simulink model "Simulink_AcraV3"  (R2018a)
settings: Solver=VariableStepAuto  StartTime=0.0  StopTime=total_time  FixedStep=step  RelTol=1e-3  AbsTol=1e-3  EnableMultiTasking=on
values from neighbouring files (symbols this model uses):
  C1 = 35/1000    (= 0.035)    [ACRA_simulink.m]
  C2 = 32/1000    (= 0.032)    [ACRA_simulink.m]
  K_ow = 20    [ACRA_simulink.m]
  K_peep = 25    [ACRA_simulink.m]
  Kv1 = 30    [ACRA_simulink.m]
  Kv2 = 40    [ACRA_simulink.m]
  PEEP_v1 = 5    [ACRA_simulink.m]
  PEEP_v2 = 7    [ACRA_simulink.m]
  R1 = 5    [ACRA_simulink.m]
  R2 = 7    [ACRA_simulink.m]
  R_vent = 1.5    [ACRA_simulink.m]
libraries: sh_lib x23, fl_lib x16, nesl_utility x9, sdl_lib x4
settings Model: Creator=Pedro  LastModifiedBy=Pedro
settings SolverCC: AutoScaleAbsTol=off  ZeroCrossAlgorithm=Adaptive
settings DataIOCC: LimitDataPoints=on  MaxDataPoints=10000
settings OptimizationCC: LifeSpan=inf
settings DebuggingCC: IgnoredZcDiagnostic=none  AllowSymbolicDim=off  SFUnexpectedBacktrackingDiag=warning  SFNoUnconditionalDefaultTransitionDiag=warning  SFExecutionAtInitializationDiag=none
settings CodeAppCC: StateflowObjectComments=on
settings GRTTargetCC: TargetLangStandard=C89/C90 (ANSI)  GeneratePreprocessorConditionals=Disable all
settings ConfigComp: CovMetricSettings=dw  CovHtmlReporting=on  CovSaveCumulativeToWorkspaceVar=on  CovSaveSingleToWorkspaceVar=on  CovExternalEMLEnable=off  CovSFcnEnable=off
settings SimscapeCC: SimscapeLogType=all  SimscapeLogDataHistory=10000

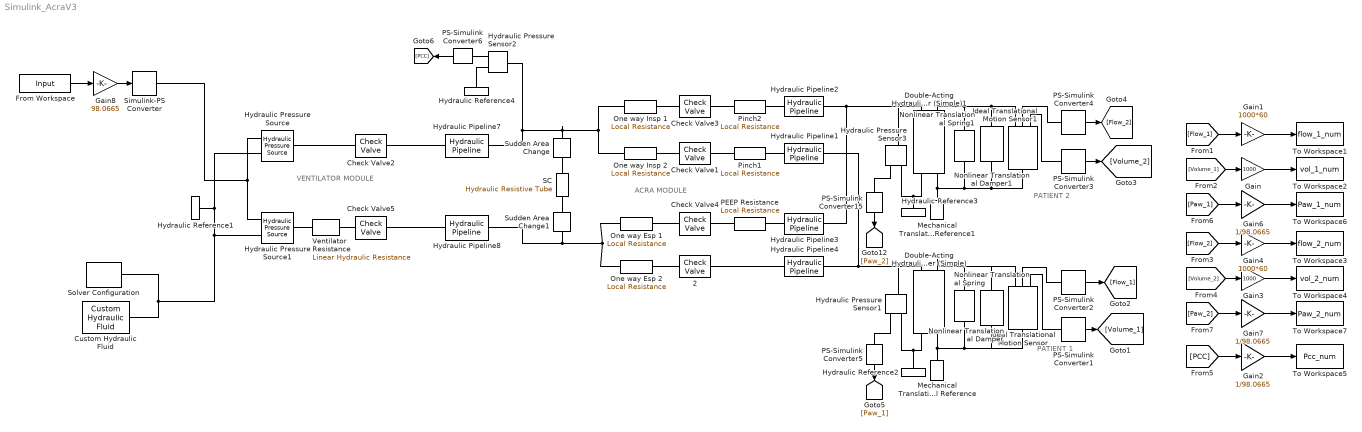
== system Simulink_AcraV3 ==
  note: PATIENT 2
  note: PATIENT 1
  note: VENTILATOR
      | MODULE
  note: ACRA MODULE
  " 2" : sh_lib/Valves/Directional Valves/Check Valve  area_max=5 cm^2  pres_crack=1 Pa  pres_max=10 Pa  C_d=1  A_leak=1e-12 cm^2  lam_spec=1  B_lam=0.999  Re_cr=12  dynamic=1  tau=0.05 s  area_init=1e-12 m^2
      settings: SourceProductName=Simscape Fluids  SourceProductBaseCode=SH
  Check Valve1 : sh_lib/Valves/Directional Valves/Check Valve  area_max=5 cm^2  pres_crack=1 Pa  pres_max=10 Pa  C_d=1  A_leak=1e-12 mm^2  lam_spec=2  B_lam=0.999  Re_cr=1000  dynamic=1  tau=0.05 s  area_init=1e-12 m^2
      settings: SourceProductName=Simscape Fluids  SourceProductBaseCode=SH
  Check Valve2 : sh_lib/Valves/Directional Valves/Check Valve  area_max=5 cm^2  pres_crack=1 Pa  pres_max=10 Pa  C_d=1  A_leak=1e-12 mm^2  lam_spec=2  B_lam=0.999  Re_cr=1000  dynamic=1  tau=0.05 s  area_init=1e-12 m^2
      settings: SourceProductName=Simscape Fluids  SourceProductBaseCode=SH
  Check Valve3 : sh_lib/Valves/Directional Valves/Check Valve  area_max=5 cm^2  pres_crack=1 Pa  pres_max=10 Pa  C_d=1  A_leak=1e-12 mm^2  lam_spec=2  B_lam=0.999  Re_cr=1000  dynamic=1  tau=0.05 s  area_init=1e-12 m^2
      settings: SourceProductName=Simscape Fluids  SourceProductBaseCode=SH
  Check Valve4 : sh_lib/Valves/Directional Valves/Check Valve  area_max=1 cm^2  pres_crack=(PEEP_v2-PEEP_v1+0.01)*98 Pa  pres_max=(PEEP_v2-PEEP_v1+0.01)*98.1 Pa  C_d=1  A_leak=1e-12 mm^2  lam_spec=2  B_lam=0.999  Re_cr=4000  dynamic=1  tau=0.05 s  area_init=1e-12 m^2
      settings: SourceProductName=Simscape Fluids  SourceProductBaseCode=SH
  Check Valve5 : sh_lib/Valves/Directional Valves/Check Valve  area_max=0.8 cm^2  pres_crack=0.01*98 Pa  pres_max=0.2*98 Pa  C_d=1  A_leak=1e-12 mm^2  lam_spec=2  B_lam=0.999  Re_cr=4000  dynamic=1  tau=0.1 s  area_init=1e-12 m^2
      settings: SourceProductName=Simscape Fluids  SourceProductBaseCode=SH
  Custom Hydraulic Fluid : fl_lib/Hydraulic/Hydraulic Utilities/Custom Hydraulic Fluid  density=1.225 kg/m^3  viscosity_kin=1.5e-5 m^2/s  bulk=142 kPa  alpha=0.005  range_error=2
      settings: SourceProductName=Foundation Library
  Double-Acting Hydraulic Cylinder (Simple) : sh_lib/Hydraulic Cylinders/Double-Acting Hydraulic Cylinder (Simple)  area_A=1 m^2  area_B=1 m^2  stroke=1 m  init_pos=0 m  penetr_coeff=1e12 s*N/m^2  or=1
      settings: SourceProductName=Simscape Fluids  SourceProductBaseCode=SH
  Double-Acting Hydraulic Cylinder (Simple)1 : sh_lib/Hydraulic Cylinders/Double-Acting Hydraulic Cylinder (Simple)  area_A=1 m^2  area_B=1 m^2  stroke=1 m  init_pos=0 m  penetr_coeff=1e12 s*N/m^2  or=1
      settings: SourceProductName=Simscape Fluids  SourceProductBaseCode=SH
  From Workspace : FromWorkspace  VariableName=Input  OutDataTypeStr=double  SampleTime=0
  Gain : Gain  Gain=1000
  Gain1 : Gain  Gain=1000*60
  Gain2 : Gain  Gain=1/98.0665
  Gain3 : Gain  Gain=1000
  Gain4 : Gain  Gain=1000*60
  Gain6 : Gain  Gain=1/98.0665
  Gain7 : Gain  Gain=1/98.0665
  Gain8 : Gain  Gain=98.0665
  Hydraulic Pipeline{1..4,7..8} (6 alike) : sh_lib/Pipelines/Hydraulic Pipeline  cs_type=1  d_in=20 mm  area=1e-4 m^2  D_h=1.12e-2 m  s_factor=64  length=1 m  length_ad=0.1 m  roughness=0.2 mm  Re_lam=2000  Re_turb=4000  wall_type=2  pr_r_coef=4e-8 m/Pa  time_const=0.01 s  k_sh=1.4  initial_pressure=0 Pa
      settings: SourceProductName=Simscape Fluids  SourceProductBaseCode=SH
  Hydraulic Pressure Sensor1 : fl_lib/Hydraulic/Hydraulic Sensors/Hydraulic Pressure Sensor
      settings: SourceProductName=Simscape
  Hydraulic Pressure Sensor2 : fl_lib/Hydraulic/Hydraulic Sensors/Hydraulic Pressure Sensor
      settings: SourceProductName=Simscape
  Hydraulic Pressure Sensor3 : fl_lib/Hydraulic/Hydraulic Sensors/Hydraulic Pressure Sensor
      settings: SourceProductName=Simscape
  Hydraulic Pressure Source : fl_lib/Hydraulic/Hydraulic Sources/Hydraulic Pressure Source
      settings: SourceProductName=Simscape  SourceProductBaseCode=SS
  Hydraulic Pressure Source1 : fl_lib/Hydraulic/Hydraulic Sources/Hydraulic Pressure Source
      settings: SourceProductName=Simscape  SourceProductBaseCode=SS
  Hydraulic Reference{1..4} (4 alike) : fl_lib/Hydraulic/Hydraulic Elements/Hydraulic Reference
      settings: SourceProductName=Foundation Library
  Ideal Translational Motion Sensor : fl_lib/Mechanical/Mechanical Sensors/Ideal Translational Motion Sensor  offset=0 m
  Ideal Translational Motion Sensor1 : fl_lib/Mechanical/Mechanical Sensors/Ideal Translational Motion Sensor  offset=0 m
  Mechanical Translational Reference : fl_lib/Mechanical/Translational Elements/Mechanical Translational Reference
  Mechanical Translational Reference1 : fl_lib/Mechanical/Translational Elements/Mechanical Translational Reference
  Nonlinear Translational Damper : sdl_lib/Couplings & Drives/Springs & Dampers/Nonlinear Translational Damper  parameterization=1  symmetry=1  coefficient_vector=[R1*98*1000, 0, 0, 0, 0] N/(m/s)  extension_coefficient_vector=[10, 0, 1, 0, .1] N/(m/s)  contraction_coefficient_vector=[100, -1, 10, 0, 0] N/(m/s)  velocity_vector=[-1, -.5, -.3, -.1, .1, .3, .5, 1] m/s  force_vector=[-100, -40, -20, -5, 5, 20, 40, 100] N  interp_method=simscape.enum.interpolation.linear  extrap_method=simscape.enum.extrapolation.linear
      settings: SourceProductName=Simscape Driveline  SourceProductBaseCode=LD
  Nonlinear Translational Damper1 : sdl_lib/Couplings & Drives/Springs & Dampers/Nonlinear Translational Damper  parameterization=1  symmetry=1  coefficient_vector=[R2*98*1000, 0, 0, 0, 0] N/(m/s)  extension_coefficient_vector=[10, 0, 1, 0, .1] N/(m/s)  contraction_coefficient_vector=[100, -1, 10, 0, 0] N/(m/s)  velocity_vector=[-1, -.5, -.3, -.1, .1, .3, .5, 1] m/s  force_vector=[-100, -40, -20, -5, 5, 20, 40, 100] N  interp_method=simscape.enum.interpolation.linear  extrap_method=simscape.enum.extrapolation.linear
      settings: SourceProductName=Simscape Driveline  SourceProductBaseCode=LD
  Nonlinear Translational Spring : sdl_lib/Couplings & Drives/Springs & Dampers/Nonlinear Translational Spring  parameterization=1  symmetry=1  coefficient_vector=[1000*98.0665/C1, 0, 0, 0, 0] N/m  tension_coefficient_vector=[100, 0, 10, 0, 1] N/m  compression_coefficient_vector=[1000, -10, 100, 0, 0] N/m  deformation_vector=[0,100,200,400,600,800,1000,1200]*1/1000 mm  force_vector=[0,345,780,1340,1530,1600,1710,2900]*1.1 N  interp_method=simscape.enum.interpolation.linear  extrap_method=simscape.enum.extrapolation.linear  x_specify=off  x_priority=High  x=0 m  x_nominal_specify=off  x_nominal_unit=m  x_nominal_value=1
      settings: SourceProductName=Simscape Driveline  SourceProductBaseCode=LD
  Nonlinear Translational Spring1 : sdl_lib/Couplings & Drives/Springs & Dampers/Nonlinear Translational Spring  parameterization=1  symmetry=1  coefficient_vector=[1000*98.0665/C2, 0, 0, 0, 0] N/m  tension_coefficient_vector=[100, 0, 10, 0, 1] N/m  compression_coefficient_vector=[1000, -10, 100, 0, 0] N/m  deformation_vector=[0,100,200,400,600,800,1000,1200]*1/1000 mm  force_vector=[0,345,780,1340,1530,1600,1710,2900]*1.1 N  interp_method=simscape.enum.interpolation.linear  extrap_method=simscape.enum.extrapolation.linear  x_specify=off  x_priority=High  x=0 m  x_nominal_specify=off  x_nominal_unit=m  x_nominal_value=1
      settings: SourceProductName=Simscape Driveline  SourceProductBaseCode=LD
  One way Esp 1 : sh_lib/Local Hydraulic Resistances/Local Resistance  area=0.000198456 m^2  mdl_type=2  kp_d=40  kp_r=40  lam_spec=2  B_lam=0.999  Re_cr=1000  Re_vec=[-10000 , 0, 10000]  loss_coeff_vec=[1,1,1]*(K_ow)  interp_method=1  extrap_method=2  flow_rate_threshold=1e-6 m^3/s  flow_rate_specify=off  flow_rate_priority=None  flow_rate=0 m^3/s  flow_rate_nominal_specify=off  flow_rate_nominal_unit=m^3/s  flow_rate_nominal_value=1  pressure_drop_specify=off  pressure_drop_priority=None  pressure_drop=0 Pa  pressure_drop_nominal_specify=off  pressure_drop_nominal_unit=Pa  pressure_drop_nominal_value=1
      settings: SourceProductName=Simscape Fluids  SourceProductBaseCode=SH
  One way Esp 2 : sh_lib/Local Hydraulic Resistances/Local Resistance  area=0.000198456 m^2  mdl_type=2  kp_d=40  kp_r=40  lam_spec=2  B_lam=0.999  Re_cr=1000  Re_vec=[-10000 , 0, 10000]  loss_coeff_vec=[1,1,1]*K_ow  interp_method=1  extrap_method=2  flow_rate_threshold=1e-6 m^3/s  flow_rate_specify=off  flow_rate_priority=None  flow_rate=0 m^3/s  flow_rate_nominal_specify=off  flow_rate_nominal_unit=m^3/s  flow_rate_nominal_value=1  pressure_drop_specify=off  pressure_drop_priority=None  pressure_drop=0 Pa  pressure_drop_nominal_specify=off  pressure_drop_nominal_unit=Pa  pressure_drop_nominal_value=1
      settings: SourceProductName=Simscape Fluids  SourceProductBaseCode=SH
  One way Insp 1 : sh_lib/Local Hydraulic Resistances/Local Resistance  area=0.000198456 m^2  mdl_type=2  kp_d=40  kp_r=40  lam_spec=2  B_lam=0.999  Re_cr=1000  Re_vec=[-10000 , 0, 10000]  loss_coeff_vec=[1,1,1]*K_ow  interp_method=1  extrap_method=2  flow_rate_threshold=1e-6 m^3/s  flow_rate_specify=off  flow_rate_priority=None  flow_rate=0 m^3/s  flow_rate_nominal_specify=off  flow_rate_nominal_unit=m^3/s  flow_rate_nominal_value=1  pressure_drop_specify=off  pressure_drop_priority=None  pressure_drop=0 Pa  pressure_drop_nominal_specify=off  pressure_drop_nominal_unit=Pa  pressure_drop_nominal_value=1
      settings: SourceProductName=Simscape Fluids  SourceProductBaseCode=SH
  One way Insp 2 : sh_lib/Local Hydraulic Resistances/Local Resistance  area=0.000198456 m^2  mdl_type=2  kp_d=40  kp_r=40  lam_spec=2  B_lam=0.999  Re_cr=1000  Re_vec=[-10000 , 0, 10000]  loss_coeff_vec=[1,1,1]*K_ow  interp_method=1  extrap_method=2  flow_rate_threshold=1e-6 m^3/s  flow_rate_specify=off  flow_rate_priority=None  flow_rate=0 m^3/s  flow_rate_nominal_specify=off  flow_rate_nominal_unit=m^3/s  flow_rate_nominal_value=1  pressure_drop_specify=off  pressure_drop_priority=None  pressure_drop=0 Pa  pressure_drop_nominal_specify=off  pressure_drop_nominal_unit=Pa  pressure_drop_nominal_value=1
      settings: SourceProductName=Simscape Fluids  SourceProductBaseCode=SH
  PEEP Resistance : sh_lib/Local Hydraulic Resistances/Local Resistance  area=0.000198456 m^2  mdl_type=2  kp_d=40  kp_r=40  lam_spec=2  B_lam=0.999  Re_cr=1000  Re_vec=[-10000 , 0, 10000]  loss_coeff_vec=[1,1,1]*(K_peep)  interp_method=1  extrap_method=2  flow_rate_threshold=1e-6 m^3/s  flow_rate_specify=off  flow_rate_priority=None  flow_rate=0 m^3/s  flow_rate_nominal_specify=off  flow_rate_nominal_unit=m^3/s  flow_rate_nominal_value=1  pressure_drop_specify=off  pressure_drop_priority=None  pressure_drop=0 Pa  pressure_drop_nominal_specify=off  pressure_drop_nominal_unit=Pa  pressure_drop_nominal_value=1
      settings: SourceProductName=Simscape Fluids  SourceProductBaseCode=SH
  PS-Simulink Converter{1..6,15} (7 alike) : nesl_utility/PS-Simulink Converter  PhysicalDomain=network_engine_domain  SubClassName=ps_output  LeftPortType=input  RightPortType=output  PseudoPeriodic=off  Frequencies=[]  Unit=1  AffineConversion=off
  Pinch1 : sh_lib/Local Hydraulic Resistances/Local Resistance  area=0.000198456 m^2  mdl_type=2  kp_d=40  kp_r=40  lam_spec=2  B_lam=0.999  Re_cr=1000  Re_vec=[-10000 , 0, 10000]  loss_coeff_vec=[1,1,1]*Kv1  interp_method=1  extrap_method=2  flow_rate_threshold=1e-6 m^3/s  flow_rate_specify=off  flow_rate_priority=None  flow_rate=0 m^3/s  flow_rate_nominal_specify=off  flow_rate_nominal_unit=m^3/s  flow_rate_nominal_value=1  pressure_drop_specify=off  pressure_drop_priority=None  pressure_drop=0 Pa  pressure_drop_nominal_specify=off  pressure_drop_nominal_unit=Pa  pressure_drop_nominal_value=1
      settings: SourceProductName=Simscape Fluids  SourceProductBaseCode=SH
  Pinch2 : sh_lib/Local Hydraulic Resistances/Local Resistance  area=0.000198456 m^2  mdl_type=2  kp_d=40  kp_r=40  lam_spec=2  B_lam=0.999  Re_cr=1000  Re_vec=[-10000 , 0, 10000]  loss_coeff_vec=[1,1,1]*Kv2  interp_method=1  extrap_method=2  flow_rate_threshold=1e-6 m^3/s  flow_rate_specify=off  flow_rate_priority=None  flow_rate=0 m^3/s  flow_rate_nominal_specify=off  flow_rate_nominal_unit=m^3/s  flow_rate_nominal_value=1  pressure_drop_specify=off  pressure_drop_priority=None  pressure_drop=0 Pa  pressure_drop_nominal_specify=off  pressure_drop_nominal_unit=Pa  pressure_drop_nominal_value=1
      settings: SourceProductName=Simscape Fluids  SourceProductBaseCode=SH
  SC : fl_lib/Hydraulic/Hydraulic Elements/Hydraulic Resistive Tube  cs_type=1  d_in=3.5 mm  area=1e-4 m^2  D_h=1.12e-2 m  s_factor=64  length=15 cm  length_ad=0 cm  roughness=0.01 mm  Re_lam=2000  Re_turb=4000  q_specify=off  q_priority=None  q=0.001 m^3/s  q_nominal_specify=off  q_nominal_unit=m^3/s  q_nominal_value=1  p_specify=off  p_priority=None  p=0 Pa  p_nominal_specify=off  p_nominal_unit=Pa  p_nominal_value=1
      settings: SourceProductName=Simscape  SourceProductBaseCode=SS
  Simulink-PS Converter : nesl_utility/Simulink-PS Converter  PhysicalDomain=network_engine_domain  SubClassName=ps_input  LeftPortType=input  RightPortType=output  PseudoPeriodic=off  Frequencies=[]  NoiseDistribution=none  NoiseParameters=[]  Unit=Pa  AffineConversion=off  FilteringAndDerivatives=provide  SimscapeFilterOrder=1  InputFilterTimeConstant=0.001  UdotUserProvided=0
  Solver Configuration : nesl_utility/Solver Configuration  PhysicalDomain=network_engine_domain  SubClassName=solver  LeftPortType=input  RightPortType=generic  Tones=[]  Harmonics=[]  SimulateNoise=off  Profile=off  UseLocalSampling=off  EnableSwitchedLinearOptims=on  FrequencyDomain=off  UseCCode=off  RelTol=0.001  AbsTol=1e-06  MinStep=1e-09  ToWorkspace=off  RevertToSquareIcSolve=off  NumHomotopyIterations=100  PhasorMode=off  PhasorModeNumHarmonics=1  DoDC=off  ResidualTolerance=1e-09  UseLocalSolver=off  LocalSolverChoice=NE_BACKWARD_EULER_ADVANCER  LocalSolverSampleTime=step  DoFixedCost=off  MaxNonlinIter=3  MaxModeIter=2  LinearAlgebra=Sparse  EquationFormulation=NE_TIME_EF  DelaysMemoryBudget=1024  AutomaticFiltering=on  FilteringTimeConstant=0.001
  Sudden Area Change : sh_lib/Local Hydraulic Resistances/Sudden Area Change  mdl_type=1  small_diam=3.5 mm  large_diam=15 mm  kp_c=0.5  lam_spec=2  B_lam=0.999  Re_cr=1500  Re_vec=[-4000, -3000, -2000, -1000, -500, -200, -100, -50, -40, -30, -20, -15, -10, 10, 20, 30, 40, 50, 100, 200, 500, 1000, 2000, 4000, 5000, 10000]  loss_coeff_vec=[.25, .3, .65, .9, .65, .75, .9, 1.15, 1.35, 1.65, 2.3, 2.8, 3.1, 5, 2.7, 1.8, 1.46, 1.3, .9, .65, .42, .3, .2, .4, .42, .25]  interp_method=2  extrap_method=2
      settings: SourceProductName=Simscape Fluids  SourceProductBaseCode=SH
  Sudden Area Change1 : sh_lib/Local Hydraulic Resistances/Sudden Area Change  mdl_type=1  small_diam=3.5 mm  large_diam=15 mm  kp_c=0.5  lam_spec=2  B_lam=0.999  Re_cr=1500  Re_vec=[-4000, -3000, -2000, -1000, -500, -200, -100, -50, -40, -30, -20, -15, -10, 10, 20, 30, 40, 50, 100, 200, 500, 1000, 2000, 4000, 5000, 10000]  loss_coeff_vec=[.25, .3, .65, .9, .65, .75, .9, 1.15, 1.35, 1.65, 2.3, 2.8, 3.1, 5, 2.7, 1.8, 1.46, 1.3, .9, .65, .42, .3, .2, .4, .42, .25]  interp_method=2  extrap_method=2
      settings: SourceProductName=Simscape Fluids  SourceProductBaseCode=SH
  To Workspace1 : ToWorkspace  VariableName=flow_1_num  SampleTime=0.01
      settings: Save2DSignal=2-D array (concatenate along first dimension)
  To Workspace2 : ToWorkspace  VariableName=vol_1_num  SampleTime=0.01
      settings: Save2DSignal=2-D array (concatenate along first dimension)
  To Workspace3 : ToWorkspace  VariableName=flow_2_num  SampleTime=0.01
      settings: Save2DSignal=2-D array (concatenate along first dimension)
  To Workspace4 : ToWorkspace  VariableName=vol_2_num  SampleTime=0.01
      settings: Save2DSignal=2-D array (concatenate along first dimension)
  To Workspace5 : ToWorkspace  VariableName=Pcc_num  SampleTime=0.01
      settings: Save2DSignal=2-D array (concatenate along first dimension)
  To Workspace6 : ToWorkspace  VariableName=Paw_1_num  SampleTime=0.01
      settings: Save2DSignal=2-D array (concatenate along first dimension)
  To Workspace7 : ToWorkspace  VariableName=Paw_2_num  SampleTime=0.01
      settings: Save2DSignal=2-D array (concatenate along first dimension)
  Ventilator Resistance : fl_lib/Hydraulic/Hydraulic Elements/Linear Hydraulic Resistance  resistance=R_vent*98*1000 Pa/(m^3/s)  q_specify=off  q_priority=None  q=0.001 m^3/s  q_nominal_specify=off  q_nominal_unit=m^3/s  q_nominal_value=1  p_specify=off  p_priority=None  p=0 Pa  p_nominal_specify=off  p_nominal_unit=Pa  p_nominal_value=1
      settings: SourceProductName=Simscape  SourceProductBaseCode=SS
  wires:
  Gain/1 -> To Workspace2/1
  Gain1/1 -> To Workspace1/1
  [Volume_1] -> Gain/1
  [Flow_1] -> Gain1/1
  Gain3/1 -> To Workspace4/1
  [Volume_2] -> Gain3/1
  Gain4/1 -> To Workspace3/1
  [Flow_2] -> Gain4/1
  [Paw_1] -> Gain6/1
  Gain6/1 -> To Workspace6/1
  [Paw_2] -> Gain7/1
  Gain7/1 -> To Workspace7/1
  PS-Simulink Converter4/1 -> [Flow_2]
  PS-Simulink Converter2/1 -> [Flow_1]
  PS-Simulink Converter3/1 -> [Volume_2]
  PS-Simulink Converter1/1 -> [Volume_1]
  PS-Simulink Converter5/1 -> [Paw_1]
  Gain8/1 -> Simulink-PS Converter/1
  From Workspace/1 -> Gain8/1
  PS-Simulink Converter15/1 -> [Paw_2]
  PS-Simulink Converter6/1 -> [PCC]
  [PCC] -> Gain2/1
  Gain2/1 -> To Workspace5/1
  connections:
  Double-Acting Hydraulic Cylinder (Simple)/LConn1 -- Ideal Translational Motion Sensor/RConn1 -- Nonlinear Translational Damper/RConn1 -- Nonlinear Translational Spring/RConn1
  Double-Acting Hydraulic Cylinder (Simple)/RConn1 -- Ideal Translational Motion Sensor/LConn1 -- Nonlinear Translational Damper/LConn1 -- Nonlinear Translational Spring/LConn1 -- Mechanical Translational Reference/LConn1
  Hydraulic Reference1/LConn1 -- Hydraulic Pressure Source1/RConn2 -- Solver Configuration/RConn1 -- Custom Hydraulic Fluid/RConn1 -- Hydraulic Pressure Source/RConn2
  Ideal Translational Motion Sensor/RConn3 -- PS-Simulink Converter1/LConn1
  Ideal Translational Motion Sensor/RConn2 -- PS-Simulink Converter2/LConn1
  Double-Acting Hydraulic Cylinder (Simple)/RConn2 -- Hydraulic Pressure Sensor1/RConn1 -- Hydraulic Reference2/LConn1
  Hydraulic Reference3/LConn1 -- Hydraulic Pressure Sensor3/RConn1 -- Double-Acting Hydraulic Cylinder (Simple)1/RConn2
  Ideal Translational Motion Sensor1/RConn1 -- Nonlinear Translational Damper1/RConn1 -- Nonlinear Translational Spring1/RConn1 -- Double-Acting Hydraulic Cylinder (Simple)1/LConn1
  Ideal Translational Motion Sensor1/LConn1 -- Nonlinear Translational Damper1/LConn1 -- Nonlinear Translational Spring1/LConn1 -- Mechanical Translational Reference1/LConn1 -- Double-Acting Hydraulic Cylinder (Simple)1/RConn1
  Ideal Translational Motion Sensor1/RConn2 -- PS-Simulink Converter4/LConn1
  Ideal Translational Motion Sensor1/RConn3 -- PS-Simulink Converter3/LConn1
  Check Valve1/LConn1 -- One way Insp 2/RConn1
  Check Valve3/LConn1 -- One way Insp 1/RConn1
  Hydraulic Pipeline1/LConn1 -- Hydraulic Pressure Sensor1/LConn1 -- Double-Acting Hydraulic Cylinder (Simple)/LConn2 -- Hydraulic Pipeline4/LConn1
  Hydraulic Pipeline2/RConn1 -- Pinch2/RConn1
  SC/LConn1 -- Sudden Area Change/RConn1
  Hydraulic Pressure Sensor3/LConn1 -- Hydraulic Pipeline3/LConn1 -- Hydraulic Pipeline2/LConn1 -- Double-Acting Hydraulic Cylinder (Simple)1/LConn2
  Check Valve4/RConn1 -- One way Esp 1/RConn1
  Hydraulic Pressure Sensor1/RConn2 -- PS-Simulink Converter5/LConn1
  Hydraulic Pressure Source/RConn1 -- Hydraulic Pressure Source1/RConn1 -- Simulink-PS Converter/RConn1
  Hydraulic Pressure Sensor3/RConn2 -- PS-Simulink Converter15/LConn1
  Hydraulic Pipeline7/RConn1 -- Check Valve2/RConn1
  Hydraulic Pipeline1/RConn1 -- Pinch1/RConn1
  One way Esp 2/RConn1 -- " 2"/RConn1
  Hydraulic Pipeline8/RConn1 -- Sudden Area Change1/LConn1 -- One way Esp 2/LConn1 -- One way Esp 1/LConn1
  Sudden Area Change/LConn1 -- One way Insp 2/LConn1 -- One way Insp 1/LConn1 -- Hydraulic Pressure Sensor2/LConn1 -- Hydraulic Pipeline7/LConn1
  Hydraulic Pipeline4/RConn1 -- " 2"/LConn1
  Pinch2/LConn1 -- Check Valve3/RConn1
  Pinch1/LConn1 -- Check Valve1/RConn1
  Hydraulic Pressure Source/LConn1 -- Check Valve2/LConn1
  Sudden Area Change1/RConn1 -- SC/RConn1
  PS-Simulink Converter6/LConn1 -- Hydraulic Pressure Sensor2/RConn2
  Ventilator Resistance/LConn1 -- Check Valve5/RConn1
  Check Valve5/LConn1 -- Hydraulic Pipeline8/LConn1
  Ventilator Resistance/RConn1 -- Hydraulic Pressure Source1/LConn1
  PEEP Resistance/RConn1 -- Hydraulic Pipeline3/RConn1
  Check Valve4/LConn1 -- PEEP Resistance/LConn1
  Hydraulic Pressure Sensor2/RConn1 -- Hydraulic Reference4/LConn1
